simulink model "vexv5_Clawbot_VRC_Template"  (R2019a)
settings: Solver=FixedStepDiscrete  StartTime=0.0  StopTime=Inf  RelTol=1e-3  EnableMultiTasking=on
libraries: vexv5lib x13, vexcommonlib x1
settings Model: Creator=The MathWorks, Inc.  LastModifiedBy=josea
settings DataIOCC: LimitDataPoints=on  SaveFormat=Array  ReturnWorkspaceOutputs=off
settings OptimizationCC: DefaultUnderspecifiedDataType=single  LifeSpan=1  MaxStackSize=64
settings DebuggingCC: SolverPrmCheckMsg=warning  AllowSymbolicDim=off  SFUnexpectedBacktrackingDiag=warning  SFNoUnconditionalDefaultTransitionDiag=warning  SFExecutionAtInitializationDiag=none  ArithmeticOperatorsInVariantConditions=warning
settings HardwareCC: ProdBitPerPointer=32  ProdBitPerSizeT=32  ProdBitPerPtrDiffT=32  ProdLargestAtomicInteger=Long  ProdLargestAtomicFloat=Double  ProdWordSize=32  ProdHWDeviceType=ARM Compatible->ARM Cortex  UseEmbeddedCoderFeatures=off
settings ModelReferenceCC: PropagateSignalLabelsOutOfModel=off
settings SFSimCC: SimUseLocalCustomCode=off
settings RTWCC: SystemTargetFile=ert.tlc  HardwareBoard=VEX V5 Robot Brain  TemplateMakefile=ert_default_tmf  GenerateReport=on  RTWUseLocalCustomCode=off  Toolchain=GNU Tools for ARM Embedded Processors  LaunchReport=on
settings CodeAppCC: ForceParamTrailComments=on  OperatorAnnotations=on  StateflowObjectComments=on  MATLABSourceComments=on
settings ERTTargetCC: MultiwordLength=2048  ERTCustomFileBanners=off  SupportContinuousTime=on  SupportNonInlinedSFcns=on  RemoveResetFunc=off  ModelStepFunctionPrototypeControlCompliant=off
settings ConfigComp: CovMetricSettings=dw  CovHtmlReporting=on  CovSaveCumulativeToWorkspaceVar=on  CovSaveSingleToWorkspaceVar=on  CovExternalEMLEnable=off  CovSFcnEnable=off

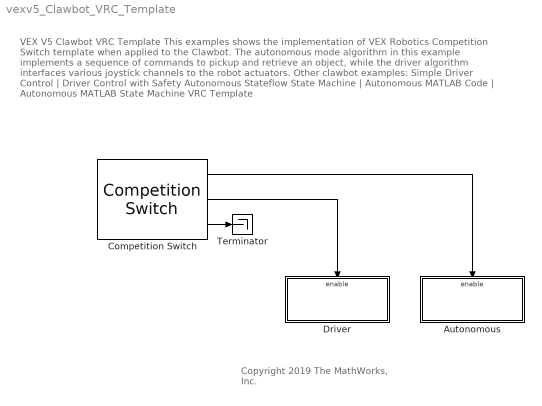
== system vexv5_Clawbot_VRC_Template ==
  note: Copyright 2019 The MathWorks, Inc.
  note: VEX V5 Clawbot VRC Template
      | This examples shows the implementation of VEX Robotics Competition Switch template when applied to the Clawbot.
      | The autonomous mode algorithm in this example implements a sequence of commands to pickup and retrieve
      | an object, while the driver algorithm interfaces various joystick channels to the robot actuators. Other clawbot examples:
      | Simple Driver Control | Driver Control with Safety
      | Autonomous Stateflow State Machine | Autonomous MATLAB Code | Autonomous MATLAB State Machine
      | VRC Template
  Autonomous : Subsystem  TreatAsAtomicUnit=on
  Competition Switch : vexv5lib/Gamepad/Competition Switch  SampleTime=0.02
      settings: SourceProductName=Simulink Coder Support Package for VEX EDR V5 Robot Brain  SourceProductBaseCode=VEXV5
  Driver : Subsystem  TreatAsAtomicUnit=on
  Terminator : Terminator
  wires:
  Competition Switch/1 -> Autonomous/Enable
  Competition Switch/2 -> Driver/Enable
  Competition Switch/3 -> Terminator/1

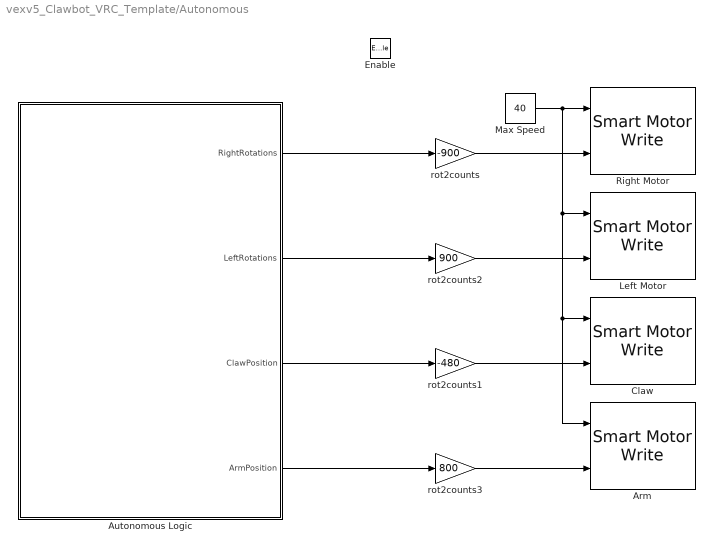
== system vexv5_Clawbot_VRC_Template/Autonomous ==
  Enable : EnablePort
  Arm : vexv5lib/Actuators/Smart Motor Write  motorPort=8  scaleFactor=18:1  MotorBrakeMode=Hold  OperationMode=Position Control
      settings: SourceProductName=Simulink Coder Support Package for VEX EDR V5 Robot Brain
  Autonomous Logic : Stateflow chart  TreatAsAtomicUnit=on
  Claw : vexv5lib/Actuators/Smart Motor Write  motorPort=3  scaleFactor=18:1  MotorBrakeMode=Hold  OperationMode=Position Control
      settings: SourceProductName=Simulink Coder Support Package for VEX EDR V5 Robot Brain
  Left Motor : vexv5lib/Actuators/Smart Motor Write  motorPort=1  scaleFactor=18:1  MotorBrakeMode=Brake  OperationMode=Position Control
      settings: SourceProductName=Simulink Coder Support Package for VEX EDR V5 Robot Brain
  Max Speed : Constant  Value=40
  Right Motor : vexv5lib/Actuators/Smart Motor Write  motorPort=10  scaleFactor=18:1  MotorBrakeMode=Brake  OperationMode=Position Control
      settings: SourceProductName=Simulink Coder Support Package for VEX EDR V5 Robot Brain
  rot2counts : Gain  Gain=-900
  rot2counts1 : Gain  Gain=-480
  rot2counts2 : Gain  Gain=900
  rot2counts3 : Gain  Gain=800
  wires:
  Autonomous Logic/1(RightRotations) -> rot2counts/1
  Max Speed/1 -> Claw/1, Arm/1, Left Motor/1, Right Motor/1
  Autonomous Logic/4(ArmPosition) -> rot2counts3/1
  rot2counts1/1 -> Claw/2
  rot2counts2/1 -> Left Motor/2
  Autonomous Logic/2(LeftRotations) -> rot2counts2/1
  rot2counts3/1 -> Arm/2
  Autonomous Logic/3(ClawPosition) -> rot2counts1/1
  rot2counts/1 -> Right Motor/2

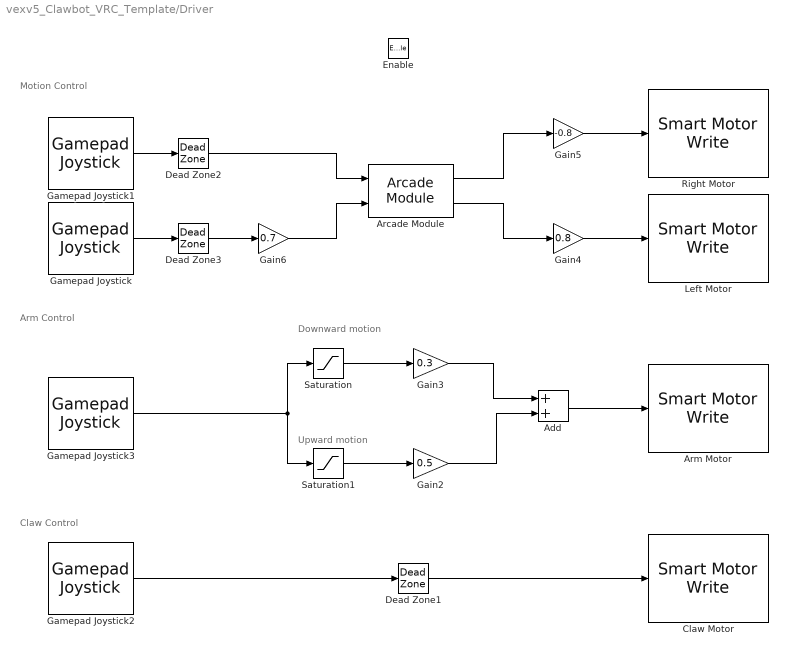
== system vexv5_Clawbot_VRC_Template/Driver ==
  note: Motion Control
  note: Arm Control
  note: Upward motion
  note: Downward motion
  note: Claw Control
  Enable : EnablePort
  Add : Sum
  Arcade Module : vexcommonlib/Arcade Module  BlockPlatform=vexarmcortex
      settings: SourceProductName=Simulink Coder Support Package for ARM Cortex-based VEX Microcontroller  SourceProductBaseCode=EC_VEX_MICRO
  Arm Motor : vexv5lib/Actuators/Smart Motor Write  motorPort=8  scaleFactor=18:1  MotorBrakeMode=Hold  OperationMode=Velocity Control
      settings: SourceProductName=Simulink Coder Support Package for VEX EDR V5 Robot Brain
  Claw Motor : vexv5lib/Actuators/Smart Motor Write  motorPort=3  scaleFactor=18:1  MotorBrakeMode=Hold  OperationMode=Velocity Control
      settings: SourceProductName=Simulink Coder Support Package for VEX EDR V5 Robot Brain
  Dead Zone1 : DeadZone  LowerValue=-5  UpperValue=5  SaturateOnIntegerOverflow=on
  Dead Zone2 : DeadZone  LowerValue=-5  UpperValue=5  SaturateOnIntegerOverflow=on
  Dead Zone3 : DeadZone  LowerValue=-5  UpperValue=5  SaturateOnIntegerOverflow=on
  Gain2 : Gain  Gain=0.5
  Gain3 : Gain  Gain=0.3
  Gain4 : Gain  Gain=0.8
  Gain5 : Gain  Gain=-0.8
  Gain6 : Gain  Gain=0.7
  Gamepad Joystick : vexv5lib/Gamepad/Gamepad Joystick  joystickType=Master  chan=4  SampleTime=0.02
      settings: SourceProductName=Simulink Coder Support Package for VEX EDR V5 Robot Brain
  Gamepad Joystick1 : vexv5lib/Gamepad/Gamepad Joystick  joystickType=Master  chan=3  SampleTime=0.02
      settings: SourceProductName=Simulink Coder Support Package for VEX EDR V5 Robot Brain
  Gamepad Joystick2 : vexv5lib/Gamepad/Gamepad Joystick  joystickType=Master  chan=1  SampleTime=0.02
      settings: SourceProductName=Simulink Coder Support Package for VEX EDR V5 Robot Brain
  Gamepad Joystick3 : vexv5lib/Gamepad/Gamepad Joystick  joystickType=Master  chan=2  SampleTime=0.02
      settings: SourceProductName=Simulink Coder Support Package for VEX EDR V5 Robot Brain
  Left Motor : vexv5lib/Actuators/Smart Motor Write  motorPort=1  scaleFactor=18:1  MotorBrakeMode=Coast  OperationMode=Velocity Control
      settings: SourceProductName=Simulink Coder Support Package for VEX EDR V5 Robot Brain
  Right Motor : vexv5lib/Actuators/Smart Motor Write  motorPort=10  scaleFactor=18:1  MotorBrakeMode=Coast  OperationMode=Velocity Control
      settings: SourceProductName=Simulink Coder Support Package for VEX EDR V5 Robot Brain
  Saturation : Saturate  UpperLimit=0  LowerLimit=-127
  Saturation1 : Saturate  UpperLimit=127  LowerLimit=0
  wires:
  Saturation/1 -> Gain3/1
  Gain6/1 -> Arcade Module/2
  Dead Zone2/1 -> Arcade Module/1
  Arcade Module/2 -> Gain4/1
  Gamepad Joystick/1 -> Dead Zone3/1
  Gain4/1 -> Left Motor/1
  Dead Zone3/1 -> Gain6/1
  Arcade Module/1 -> Gain5/1
  Saturation1/1 -> Gain2/1
  Gain3/1 -> Add/1
  Gain2/1 -> Add/2
  Gamepad Joystick1/1 -> Dead Zone2/1
  Gain5/1 -> Right Motor/1
  Add/1 -> Arm Motor/1
  Gamepad Joystick3/1 -> Saturation/1, Saturation1/1
  Gamepad Joystick2/1 -> Dead Zone1/1
  Dead Zone1/1 -> Claw Motor/1

== stateflow chart vexv5_Clawbot_VRC_Template/Autonomous/Autonomous Logic ==
  state MoveForward
    en:
    RightRotations=2;
    LeftRotations=2;
  state GrabObject
    en:
    ClawPosition=0;
  state LiftObject
    en:
    ArmPosition=1;
  state TurnAround
    en:
    RightRotations=RightRotations+1.5;
    LeftRotations=LeftRotations-1.5;
  state MoveBackward
    en:
    RightRotations=RightRotations+2;
    LeftRotations=LeftRotations+2;
  state DropObject
    en:
    ArmPosition=0;
    ClawPosition=1;
  (default) -> MoveForward : {ClawPosition=1;
      | ArmPosition=0;}
  MoveForward -> GrabObject : after(4,sec)
  GrabObject -> LiftObject : after(0.5,sec)
  LiftObject -> TurnAround : after(0.5,sec)
  TurnAround -> MoveBackward : after(4,sec)
  MoveBackward -> DropObject : after(4,sec)
  data: RightRotations output; LeftRotations output; ClawPosition output; ArmPosition output
